simulink model "InductionCoockerStateFlow"  (R2023a)
settings: Solver=FixedStepDiscrete  StartTime=0.0  StopTime=100  FixedStep=0.1  RelTol=1e-3  EnableMultiTasking=on
settings Model: Creator=antonio  LastModifiedBy=anton
settings SolverCC: AlgebraicLoopSolver=TrustRegion  AutoInsertRateTranBlk=on
settings DataIOCC: LimitDataPoints=on
settings OptimizationCC: LifeSpan=inf
settings DebuggingCC: UnconnectedInputMsg=warning  UnconnectedOutputMsg=warning  UnconnectedLineMsg=warning  AllowSymbolicDim=off  SFUnexpectedBacktrackingDiag=warning  SFNoUnconditionalDefaultTransitionDiag=warning  SFExecutionAtInitializationDiag=none  ArithmeticOperatorsInVariantConditions=warning
settings ModelReferenceCC: EnableRefExpFcnMdlSchedulingChecks=on
settings SFSimCC: SimUseLocalCustomCode=off  CustomCodeUndefinedFunction=UseInterfaceOnly
settings RTWCC: RTWUseLocalCustomCode=off  DLArmComputeVersion=19.05
settings CodeAppCC: StateflowObjectComments=on
settings GRTTargetCC: TargetLangStandard=C89/C90 (ANSI)
settings ConfigComp: CovMetricSettings=dw  CovSaveCumulativeToWorkspaceVar=on  CovSaveSingleToWorkspaceVar=on  CovExternalEMLEnable=off  CovSFcnEnable=off

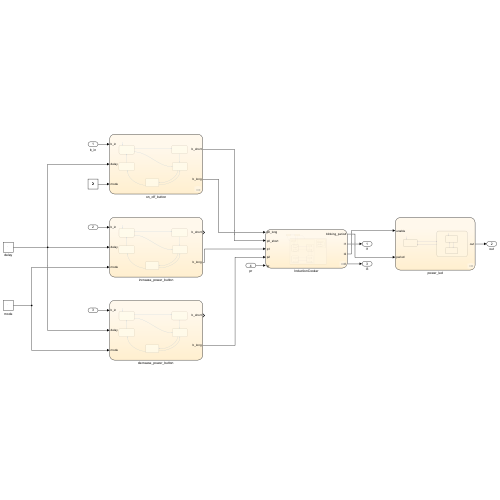
[thumbnail: Simulink's stored preview of the top-level diagram]
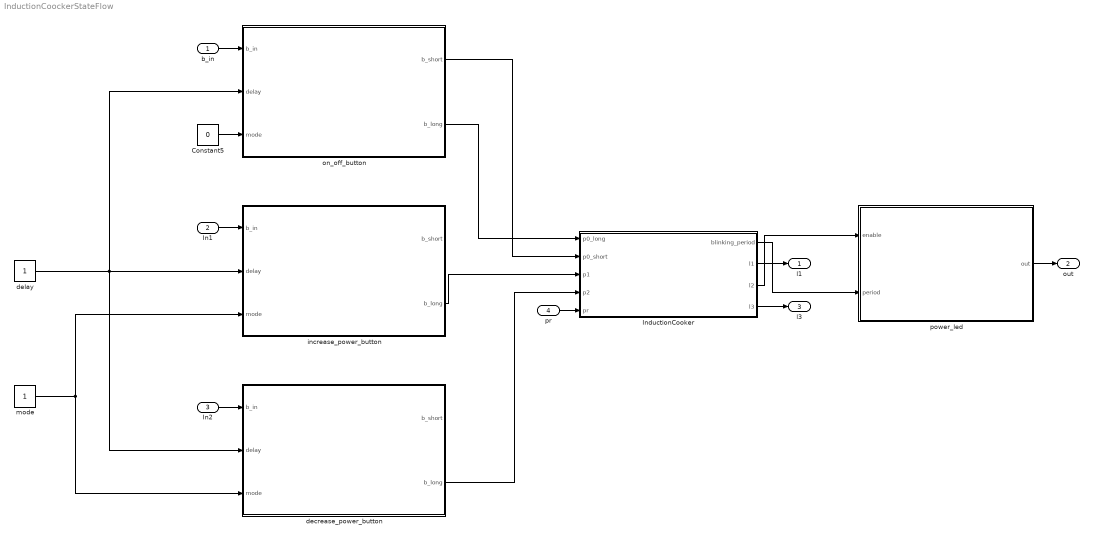
== system InductionCoockerStateFlow ==
  b_in : Inport
  In1 : Inport  Port=2
  In2 : Inport  Port=3
  pr : Inport  Port=4
  Constant5 : Constant  Value=0  OutDataTypeStr=uint8
  InductionCooker : Stateflow chart  TreatAsAtomicUnit=on
  "decrease_power_button " : Stateflow chart  TreatAsAtomicUnit=on
  delay : Constant  OutDataTypeStr=double
  increase_power_button : Stateflow chart  TreatAsAtomicUnit=on
  mode : Constant  OutDataTypeStr=uint8
  on_off_button : Stateflow chart  TreatAsAtomicUnit=on
  power_led : Stateflow chart  TreatAsAtomicUnit=on
  l1 : Outport
  out : Outport  Port=2
  l3 : Outport  Port=3
  wires:
  on_off_button/1(b_short) -> InductionCooker/2(p0_short)
  on_off_button/2(b_long) -> InductionCooker/1(p0_long)
  increase_power_button/2(b_long) -> InductionCooker/3(p1)
  "decrease_power_button "/2(b_long) -> InductionCooker/4(p2)
  InductionCooker/1(blinking_period) -> power_led/2(period)
  InductionCooker/3(l2) -> power_led/1(enable)
  InductionCooker/2(l1) -> l1/1
  Constant5/1 -> on_off_button/3(mode)
  mode/1 -> increase_power_button/3(mode), "decrease_power_button "/3(mode)
  delay/1 -> "decrease_power_button "/2(delay), increase_power_button/2(delay), on_off_button/2(delay)
  b_in/1 -> on_off_button/1(b_in)
  In1/1 -> increase_power_button/1(b_in)
  In2/1 -> "decrease_power_button "/1(b_in)
  pr/1 -> InductionCooker/5(pr)
  power_led/1(out) -> out/1
  InductionCooker/4(l3) -> l3/1

== stateflow chart InductionCoockerStateFlow/power_led ==
  state blink
    state blink_on
      en: out = ACTIVE
    state blink_off
      en: out = DISACTIVE
    (default) -> blink_on
    blink_off -> blink_on : after(period, msec)
    blink_on -> blink_off : after(period, msec)
  state off
    en: out = DISACTIVE;
  (default) -> off
  off -> blink : [enable == ACTIVE]
  blink -> off : [enable == DISACTIVE]
  data: enable input boolean; out output boolean; ACTIVE constant boolean =true; DISACTIVE constant boolean =false; period input uint32

== stateflow chart InductionCoockerStateFlow/decrease_power_button  ==
  state wait_pressed
    en: b_short = RELEASED;
    b_long = RELEASED
  state pressed
    en: b_short = PRESSED
  state wait_longpressed
    en: b_short = RELEASED
  state wait_released
    en: b_long = RELEASED
  state longpressed
    on after(delay, sec):
    b_long = PRESSED;
  (default) -> wait_pressed
  wait_pressed -> pressed [order 1] : [mode == 0 & b_in == PRESSED]
  wait_pressed -> wait_longpressed [order 2] : [mode == 1]
  pressed -> wait_longpressed : [b_in == RELEASED]
  wait_released -> wait_pressed : [b_in == RELEASED]
  longpressed -> wait_released [order 1] : [b_long == PRESSED & b_in == PRESSED]
  wait_longpressed -> longpressed : [b_in == PRESSED]
  longpressed -> wait_longpressed [order 2] : [b_in == RELEASED]
  data: b_in input boolean; delay input double; b_short output boolean; b_long output boolean; PRESSED constant boolean =false; RELEASED constant boolean =true; mode input uint8

== stateflow chart InductionCoockerStateFlow/increase_power_button ==
  state wait_pressed
    en: b_short = RELEASED;
    b_long = RELEASED
  state pressed
    en: b_short = PRESSED
  state wait_longpressed
    en: b_short = RELEASED
  state wait_released
    en: b_long = RELEASED
  state longpressed
    on after(delay, sec):
    b_long = PRESSED;
  (default) -> wait_pressed
  wait_pressed -> pressed [order 1] : [mode == 0 & b_in == PRESSED]
  wait_pressed -> wait_longpressed [order 2] : [mode == 1]
  pressed -> wait_longpressed : [b_in == RELEASED]
  wait_released -> wait_pressed : [b_in == RELEASED]
  longpressed -> wait_released [order 1] : [b_long == PRESSED & b_in == PRESSED]
  wait_longpressed -> longpressed : [b_in == PRESSED]
  longpressed -> wait_longpressed [order 2] : [b_in == RELEASED]
  data: b_in input boolean; delay input double; b_short output boolean; b_long output boolean; PRESSED constant boolean =false; RELEASED constant boolean =true; mode input uint8

== stateflow chart InductionCoockerStateFlow/on_off_button ==
  state wait_pressed
    en: b_short = RELEASED;
    b_long = RELEASED
  state pressed
    en: b_short = PRESSED
  state wait_longpressed
    en: b_short = RELEASED
  state wait_released
    en: b_long = RELEASED
  state longpressed
    on after(delay, sec):
    b_long = PRESSED;
  (default) -> wait_pressed
  wait_pressed -> pressed [order 1] : [mode == 0 & b_in == PRESSED]
  wait_pressed -> wait_longpressed [order 2] : [mode == 1]
  pressed -> wait_longpressed : [b_in == RELEASED]
  wait_released -> wait_pressed : [b_in == RELEASED]
  longpressed -> wait_released [order 1] : [b_long == PRESSED & b_in == PRESSED]
  wait_longpressed -> longpressed : [b_in == PRESSED]
  longpressed -> wait_longpressed [order 2] : [b_in == RELEASED]
  data: b_in input boolean; delay input double; b_short output boolean; b_long output boolean; PRESSED constant boolean =false; RELEASED constant boolean =true; mode input uint8

== stateflow chart InductionCoockerStateFlow/InductionCooker ==
  state off
    en: l1 = OFF; l2 = OFF, l3 = OFF,
    blinking_period = 0;
  state inactive
    en: l1 = ON; l2 = OFF; err_status = ~ERR,
    blinking_period = 0;
  state active
    state powers [parallel]
      settings: executionOrder=1
      state waiting_inactive
      state power_500w
        state waiting_500w
        state working_500w
          en: l2 = ON;
          blinking_period = DELAY_500;
        (default) -> waiting_500w
        waiting_500w -> working_500w : after(POWER_DELAY, sec)[pr == POT_IS_PRESENT]
      state power_300w
        state waiting_300w
        state working_300w
          en: l2 = ON;
          blinking_period = DELAY_300;
        (default) -> waiting_300w
        waiting_300w -> working_300w : after(POWER_DELAY, sec)[pr == POT_IS_PRESENT]
      state power_1500w
        state waiting_1500w
        state working_1500w
          en: l2 = ON;
          blinking_period = DELAY_1500;
        (default) -> waiting_1500w
        waiting_1500w -> working_1500w : after(POWER_DELAY, sec)[pr == POT_IS_PRESENT]
      state power_1000w
        state waiting_1000w
        state working_1000w
          en: l2 = ON;
          blinking_period = DELAY_1000;
        (default) -> waiting_1000w
        waiting_1000w -> working_1000w : after(POWER_DELAY, sec)[pr == POT_IS_PRESENT]
      power_300w -> waiting_inactive [order 1] : [p2 == PRESSED & pr == POT_IS_PRESENT]
      waiting_inactive -> power_300w [order 1] : [p1 == PRESSED & pr == POT_IS_PRESENT]
      (default) -> power_300w
      power_300w -> power_500w [order 2] : [p1 == PRESSED & pr == POT_IS_PRESENT]
      power_500w -> power_300w [order 1] : [p2 == PRESSED & pr == POT_IS_PRESENT]
      power_1000w -> power_500w [order 1] : [p2 == PRESSED & pr == POT_IS_PRESENT]
      power_500w -> power_1000w [order 2] : [p1 == PRESSED & pr == POT_IS_PRESENT]
      power_1500w -> power_1000w : [p2 == PRESSED & pr == POT_IS_PRESENT]
      power_1000w -> power_1500w [order 2] : [p1 == PRESSED & pr == POT_IS_PRESENT]
    state anomaly_guard [parallel]
      settings: executionOrder=2
      state guard
      state anomaly_detected
        en: l3 = ON
        exit: l3 = OFF
      (default) -> guard
      anomaly_detected -> guard [order 2] : after(ANOMALY_DELAY, sec){err_status = ERR}
      anomaly_detected -> guard [order 1] : [pr == POT_IS_PRESENT]
      guard -> anomaly_detected : [pr == ~POT_IS_PRESENT]
  (default) -> off
  off -> inactive : [p0_short == PRESSED]
  active -> inactive [order 1] : [err_status == ERR]
  inactive -> off [order 1] : [p0_long == PRESSED]
  active -> off [order 2] : [p0_long == PRESSED]
  waiting_inactive -> inactive [order 2] : after(POWER_DELAY, sec)
  inactive -> power_300w [order 2] : [p1 == PRESSED & pr == POT_IS_PRESENT]
  data: ERR constant boolean =true; DELAY_300 constant uint32 =2000; p0_long input boolean; p0_short input boolean; p1 input boolean; p2 input boolean; pr input boolean; blinking_period output uint32; l1 output boolean; l2 output boolean; l3 output boolean; err_status local boolean; ANOMALY_DELAY constant uint16 =10; DELAY_1000 constant uint32 =500; DELAY_1500 constant uint32 =250; DELAY_500 constant uint32 =1000; OFF constant boolean =false; ON constant boolean =true; POT_IS_PRESENT constant boolean =false; PRESSED constant boolean =false; POWER_DELAY constant uint16 =5
